simulink model "7step_CHBinverter_phaseshiftedSPWM"  (R2025a)
settings: Solver=FixedStepDiscrete  StartTime=0.0  StopTime=3/50  FixedStep=20e-6  RelTol=1e-3
libraries: spsMosfetLib x12, spsDCVoltageSourceLib x3, spsTriangleGeneratorLib x3, dspstat3 x1, spsSeriesRLCBranchLib x1, spsVoltageMeasurementLib x1, sps_lib x1
settings Model: Creator=ASUS  LastModifiedBy=ASUS
settings DataIOCC: SaveFinalState=on  SaveFormat=Array  SaveState=on  ReturnWorkspaceOutputs=off  LoggingToFile=on

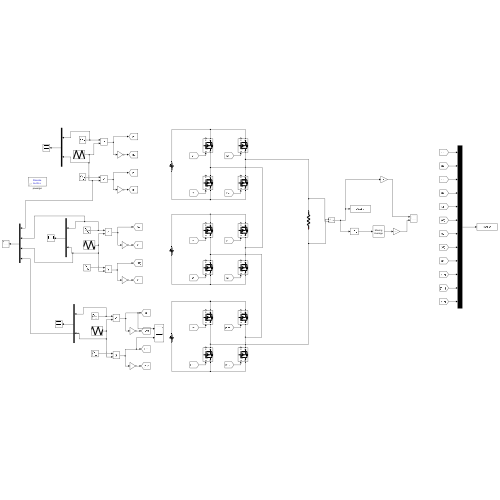
[thumbnail: Simulink's stored preview of the top-level diagram]
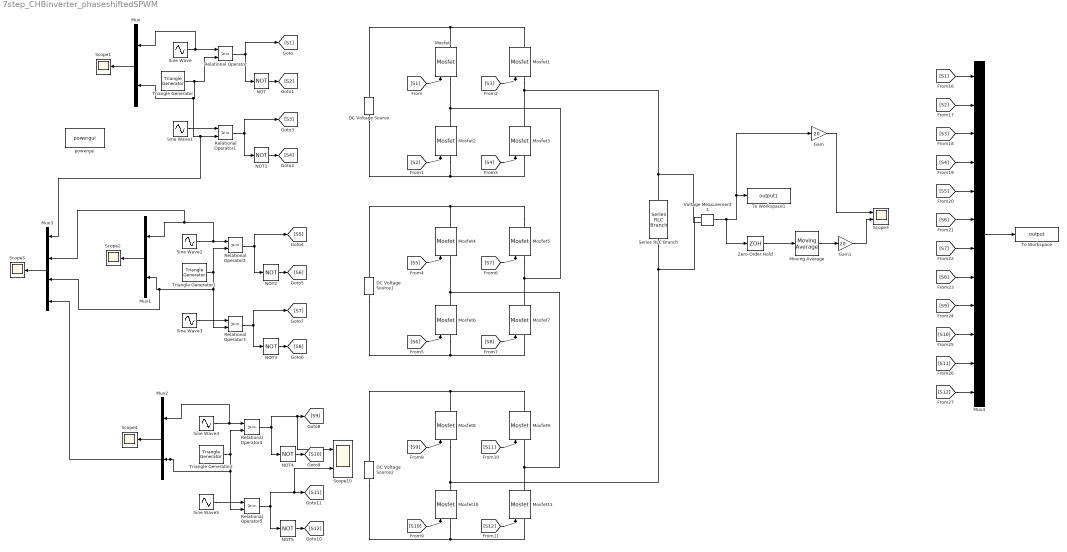
== system 7step_CHBinverter_phaseshiftedSPWM ==
  DC Voltage Source : spsDCVoltageSourceLib/DC Voltage Source  Amplitude=20  Measurements=Voltage
  DC Voltage Source1 : spsDCVoltageSourceLib/DC Voltage Source  Amplitude=20  Measurements=Voltage
  DC Voltage Source2 : spsDCVoltageSourceLib/DC Voltage Source  Amplitude=20  Measurements=Voltage
  Gain : Gain  Gain=20
  Gain1 : Gain  Gain=20
  Mosfet{,1..11} (12 alike) : spsMosfetLib/Mosfet  Ron=0.1  Lon=0  Rd=0.01  Vfd=0  IC=0  Rs=1e5  Cs=inf  Measurements=on
  Moving Average : dspstat3/Moving Average  Method=Sliding window  ForgettingFactorPort=off  SpecifyWindowLength=on  WindowLength=100  OverlapLength=99  AllowArbitraryInputLength=off  ForgettingFactor=0.9  SimulateUsing=Interpreted execution
  Mux : Mux  Inputs=2
  Mux1 : Mux  Inputs=2
  Mux2 : Mux  Inputs=2
  Mux3 : Mux
  Mux4 : Mux  Inputs=12
  NOT{,1..5} (6 alike) : Logic  Operator=NOT  IconShape=distinctive  AllPortsSameDT=off  OutDataTypeStr=boolean
  Relational Operator{,1..5} (6 alike) : RelationalOperator  OutDataTypeStr=boolean  RndMeth=Simplest  InputSameDT=off
  Scope{1..2,4..5} (4 alike) : Scope
      Scope1 settings: ActiveDisplayYMinimum=-1.25  ActiveDisplayYMaximum=1.25
      Scope2 settings: ActiveDisplayYMinimum=-1.0375354107648724  ActiveDisplayYMaximum=1.0310434372049102  DataLoggingVariableName=ScopeData2
      Scope4 settings: ActiveDisplayYMinimum=-0.99667426376371937  ActiveDisplayYMaximum=1.1675955722834359
      Scope5 settings: ActiveDisplayYMinimum=-1.1874543952270586  ActiveDisplayYMaximum=1.520194866512147  DataLoggingVariableName=ScopeData4
  Scope10 : Scope  NumInputPorts=2
      settings: ActiveDisplayYMinimum=-0.026354204096298961  ActiveDisplayYMaximum=1.9809929072474184  DataLoggingVariableName=ScopeData10
  Scope3 : Scope  NumInputPorts=2
      settings: ActiveDisplayYMinimum=-71.387771731315041  ActiveDisplayYMaximum=71.387771520047437  DataLoggingVariableName=ScopeData3
  Series RLC Branch : spsSeriesRLCBranchLib/Series RLC Branch  LConnTagsString=__new0  RConnTagsString=__new0  BranchType=R  Resistance=50  Inductance=1e-3  SetiL0=off  InitialCurrent=0  Capacitance=1e-6  Setx0=off  InitialVoltage=0  Measurements=Branch voltage
  Sine Wave : Sin  Frequency=2*pi*50  SampleTime=0
  Sine Wave1 : Sin  Amplitude=-1  Frequency=2*pi*50  SampleTime=0
  Sine Wave2 : Sin  Frequency=2*pi*50  SampleTime=0
  Sine Wave3 : Sin  Amplitude=-1  Frequency=2*pi*50  SampleTime=0
  Sine Wave4 : Sin  Frequency=2*pi*50  SampleTime=0
  Sine Wave5 : Sin  Amplitude=-1  Frequency=2*pi*50  SampleTime=0
  To Workspace : ToWorkspace  VariableName=output  SampleTime=20e-6
      settings: Save2DSignal=2-D array (concatenate along first dimension)
  To Workspace1 : ToWorkspace  VariableName=output1  SaveFormat=Structure With Time  SampleTime=20e-6
  Triangle Generator : spsTriangleGeneratorLib/Triangle Generator  Freq=1e3  Phase=0  Ts=20e-6
  Triangle Generator1 : spsTriangleGeneratorLib/Triangle Generator  Freq=1e3  Phase=60  Ts=20e-6
  Triangle Generator2 : spsTriangleGeneratorLib/Triangle Generator  Freq=1e3  Phase=120  Ts=20e-6
  Voltage Measurement1 : spsVoltageMeasurementLib/Voltage Measurement  PhasorSimulation=off  OutputType=Complex  PSBequivalent=0
  Zero-Order Hold : ZeroOrderHold  SampleTime=20e-6
  powergui : sps_lib/powergui  Priority=1  SimulationMode=Discrete  SampleTime=20e-6  frequency=60  Iterations=50  frequencyindice=0  Pbase=100e6  ErrMax=1e-4  UnitsV=kV  UnitsW=MW  buscounter=0  FunctionMessages=off  echomessages=off  EnableUseOfTLC=off  CurrentSourceSwitches=off  DisableSnubberDevices=off  DisableRonSwitches=off  DisableVfSwitches=off  DisplayEquations=off  AutomaticDiscreteSolvers=off  SolverType=Tustin/Backward Euler (TBE)  Interpol=off  ExternalGateDelay=off  methode=off  Ts=100  x0status=blocks  SPID=on  SwTol=0  HookPort=off  NonlinearTolerance=1e-4  nMaxIteration=100  ContinueOnMaxIteration=off  RestoreLinks=warning  ResistiveCurrentMeasurement=off  Frange=[0:2:500]  Ylog=off  Xlog=on  ShowGrid=off  save=off  variable=ZData  structure=0  ZoomFFT=off  StartTime=0.0  cycles=1  DisplayStyle=1  fundamental=60  FreqAxis=off  MaxFrequency=1000  frequencyindicesteady=1  RmsSteady=1  display=off
  wires:
  Mux/1 -> Scope1/1
  Sine Wave/1 -> Relational Operator/1, Mux/1
  Triangle Generator/1 -> Relational Operator/2, Mux3/1, Relational Operator1/2, Mux/2
  Relational Operator/1 -> [S1], NOT/1
  NOT/1 -> [S2]
  [S1] -> Mosfet/1
  [S2] -> Mosfet2/1
  [S4] -> Mosfet3/1
  [S3] -> Mosfet1/1
  Sine Wave1/1 -> Relational Operator1/1
  NOT1/1 -> [S4]
  [S5] -> Mosfet4/1
  [S6] -> Mosfet6/1
  [S7] -> Mosfet5/1
  [S8] -> Mosfet7/1
  NOT2/1 -> [S6]
  Mux1/1 -> Scope2/1
  Relational Operator2/1 -> [S5], NOT2/1
  NOT3/1 -> [S8]
  Relational Operator3/1 -> [S7], NOT3/1
  Relational Operator1/1 -> NOT1/1, [S3]
  Triangle Generator1/1 -> Mux3/3, Mux1/2, Relational Operator3/2, Relational Operator2/2
  Voltage Measurement1/1 -> Zero-Order Hold/1, Gain/1, To Workspace1/1
  Sine Wave3/1 -> Relational Operator3/1
  Sine Wave2/1 -> Mux3/2, Mux1/1, Relational Operator2/1
  [S9] -> Mosfet8/1
  [S10] -> Mosfet10/1
  [S11] -> Mosfet9/1
  [S12] -> Mosfet11/1
  Sine Wave5/1 -> Relational Operator5/1
  Relational Operator4/1 -> Scope10/1, [S9], NOT4/1
  NOT5/1 -> [S12]
  Sine Wave4/1 -> Mux2/1, Relational Operator4/1
  Mux2/1 -> Scope4/1
  NOT4/1 -> [S10]
  Relational Operator5/1 -> Scope10/2, [S11], NOT5/1
  Zero-Order Hold/1 -> Moving Average/1
  Moving Average/1 -> Gain1/1
  [S1] -> Mux4/1
  [S10] -> Mux4/10
  [S2] -> Mux4/2
  [S3] -> Mux4/3
  [S4] -> Mux4/4
  [S5] -> Mux4/5
  [S6] -> Mux4/6
  [S7] -> Mux4/7
  [S8] -> Mux4/8
  [S9] -> Mux4/9
  [S11] -> Mux4/11
  [S12] -> Mux4/12
  Mux4/1 -> To Workspace/1
  Mux3/1 -> Scope5/1
  Triangle Generator2/1 -> Mux3/4, Mux2/2, Relational Operator5/2, Relational Operator4/2
  Gain/1 -> Scope3/1
  Gain1/1 -> Scope3/2
  connections:
  Mosfet5/LConn1 -- Mosfet7/RConn1 -- Mosfet/LConn1 -- Mosfet2/RConn1
  DC Voltage Source/RConn1 -- Mosfet/RConn1 -- Mosfet1/RConn1
  DC Voltage Source/LConn1 -- Mosfet3/LConn1 -- Mosfet2/LConn1
  Mosfet6/LConn1 -- DC Voltage Source1/LConn1 -- Mosfet7/LConn1
  Mosfet5/RConn1 -- DC Voltage Source1/RConn1 -- Mosfet4/RConn1
  Series RLC Branch/RConn1 -- Voltage Measurement1/LConn2 -- Mosfet3/RConn1 -- Mosfet1/LConn1
  Mosfet11/LConn1 -- Mosfet10/LConn1 -- DC Voltage Source2/LConn1
  Mosfet8/RConn1 -- Mosfet9/RConn1 -- DC Voltage Source2/RConn1
  Mosfet4/LConn1 -- Mosfet9/LConn1 -- Mosfet11/RConn1 -- Mosfet6/RConn1
  Mosfet8/LConn1 -- Series RLC Branch/LConn1 -- Voltage Measurement1/LConn1 -- Mosfet10/RConn1
